simulink model "Exercicio2"  (R2021a)
settings: Solver=VariableStepAuto  StartTime=0.0  StopTime=10  RelTol=1e-3
settings Model: Creator=taffarel55  LastModifiedBy=taffarel55

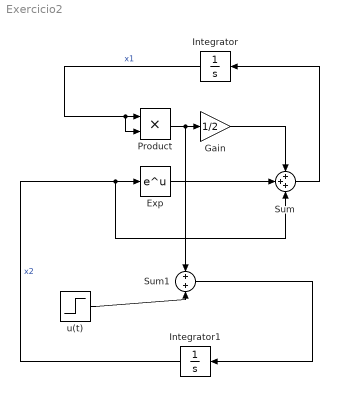
== system Exercicio2 ==
  Exp : Math  SaturateOnIntegerOverflow=on
  Gain : Gain  Gain=1/2
  Integrator : Integrator
  Integrator1 : Integrator
  Product : Product
  Sum : Sum  Inputs=+++
  Sum1 : Sum
  u(t) : Step  Time=0.8  SampleTime=0
  wires:
  Integrator/1 -> Product/2, Product/1  "x1"
  Product/1 -> Sum1/1, Gain/1
  Gain/1 -> Sum/1
  Exp/1 -> Sum/2
  Sum/1 -> Integrator/1
  u(t)/1 -> Sum1/2
  Sum1/1 -> Integrator1/1
  Integrator1/1 -> Sum/3, Exp/1  "x2"
